simulink model "BatteryPackModel"  (R2026b)
settings: Solver=VariableStepAuto
undefined symbols (not defined in the file): Battery
settings Model: DataDictionary=VehicleData.sldd  Creator=Xu Dingyi  LastModifiedBy=29358

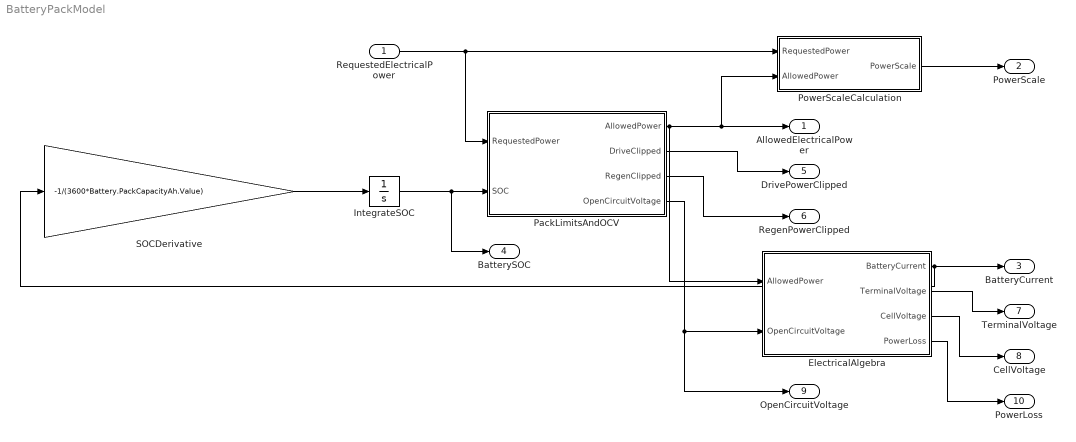
== system BatteryPackModel ==
  RequestedElectricalPower : Inport  OutDataTypeStr=double  PortDimensions=1
  ElectricalAlgebra : Subsystem
  IntegrateSOC : Integrator  InitialCondition=Battery.InitialSOC.Value  LimitOutput=on  UpperSaturationLimit=1  LowerSaturationLimit=0
  PackLimitsAndOCV : Subsystem
  PowerScaleCalculation : Subsystem
  SOCDerivative : Gain  Gain=-1/(3600*Battery.PackCapacityAh.Value)
  AllowedElectricalPower : Outport  PortDimensions=1
  PowerScale : Outport  Port=2  PortDimensions=1
  BatteryCurrent : Outport  Port=3  PortDimensions=1
  BatterySOC : Outport  Port=4  PortDimensions=1
  DrivePowerClipped : Outport  Port=5  PortDimensions=1
  RegenPowerClipped : Outport  Port=6  PortDimensions=1
  TerminalVoltage : Outport  Port=7  PortDimensions=1
  CellVoltage : Outport  Port=8  PortDimensions=1
  OpenCircuitVoltage : Outport  Port=9  PortDimensions=1
  PowerLoss : Outport  Port=10  PortDimensions=1
  wires:
  SOCDerivative/1 -> IntegrateSOC/1
  RequestedElectricalPower/1 -> PackLimitsAndOCV/1(RequestedPower), PowerScaleCalculation/1(RequestedPower)
  PackLimitsAndOCV/4(OpenCircuitVoltage) -> OpenCircuitVoltage/1, ElectricalAlgebra/2(OpenCircuitVoltage)
  PackLimitsAndOCV/3(RegenClipped) -> RegenPowerClipped/1
  PackLimitsAndOCV/2(DriveClipped) -> DrivePowerClipped/1
  PackLimitsAndOCV/1(AllowedPower) -> PowerScaleCalculation/2(AllowedPower), AllowedElectricalPower/1, ElectricalAlgebra/1(AllowedPower)
  IntegrateSOC/1 -> BatterySOC/1, PackLimitsAndOCV/2(SOC)
  PowerScaleCalculation/1(PowerScale) -> PowerScale/1
  ElectricalAlgebra/4(PowerLoss) -> PowerLoss/1
  ElectricalAlgebra/1(BatteryCurrent) -> SOCDerivative/1, BatteryCurrent/1
  ElectricalAlgebra/2(TerminalVoltage) -> TerminalVoltage/1
  ElectricalAlgebra/3(CellVoltage) -> CellVoltage/1

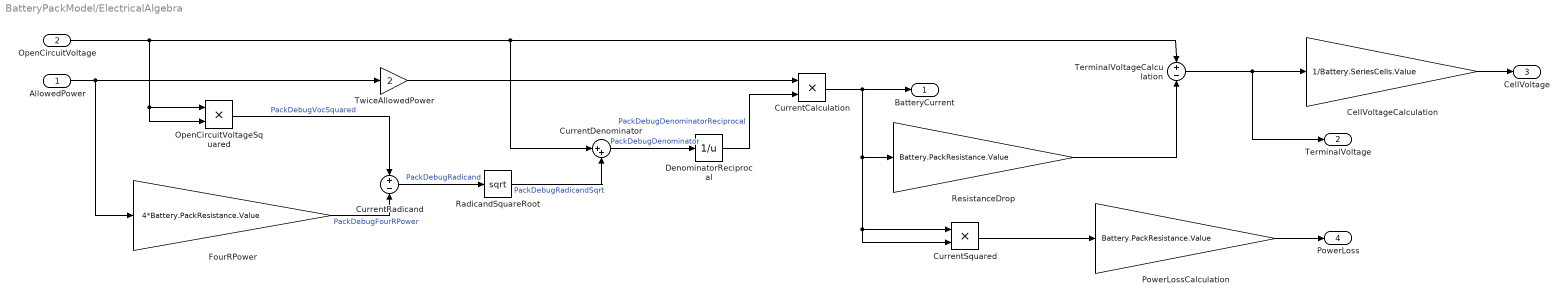
== system BatteryPackModel/ElectricalAlgebra ==
  AllowedPower : Inport
  OpenCircuitVoltage : Inport  Port=2
  CellVoltageCalculation : Gain  Gain=1/Battery.SeriesCells.Value
  CurrentCalculation : Product  Inputs=**
  CurrentDenominator : Sum  Inputs=|++
  CurrentRadicand : Sum  Inputs=+-
  CurrentSquared : Product  Inputs=**
  DenominatorReciprocal : Math  Operator=reciprocal  SignedPower=on  RndMeth=Zero
  FourRPower : Gain  Gain=4*Battery.PackResistance.Value
  OpenCircuitVoltageSquared : Product  Inputs=**
  PowerLossCalculation : Gain  Gain=Battery.PackResistance.Value
  RadicandSquareRoot : Sqrt
  ResistanceDrop : Gain  Gain=Battery.PackResistance.Value
  TerminalVoltageCalculation : Sum  Inputs=+-
  TwiceAllowedPower : Gain  Gain=2
  BatteryCurrent : Outport
  TerminalVoltage : Outport  Port=2
  CellVoltage : Outport  Port=3
  PowerLoss : Outport  Port=4
  wires:
  RadicandSquareRoot/1 -> CurrentDenominator/2  "PackDebugRadicandSqrt"
  FourRPower/1 -> CurrentRadicand/2  "PackDebugFourRPower"
  OpenCircuitVoltageSquared/1 -> CurrentRadicand/1  "PackDebugVocSquared"
  OpenCircuitVoltage/1 -> OpenCircuitVoltageSquared/2, OpenCircuitVoltageSquared/1, TerminalVoltageCalculation/1, CurrentDenominator/1
  CurrentDenominator/1 -> DenominatorReciprocal/1  "PackDebugDenominator"
  AllowedPower/1 -> TwiceAllowedPower/1, FourRPower/1
  TwiceAllowedPower/1 -> CurrentCalculation/1
  CurrentRadicand/1 -> RadicandSquareRoot/1  "PackDebugRadicand"
  DenominatorReciprocal/1 -> CurrentCalculation/2  "PackDebugDenominatorReciprocal"
  CurrentCalculation/1 -> CurrentSquared/2, CurrentSquared/1, ResistanceDrop/1, BatteryCurrent/1
  ResistanceDrop/1 -> TerminalVoltageCalculation/2
  CurrentSquared/1 -> PowerLossCalculation/1
  TerminalVoltageCalculation/1 -> TerminalVoltage/1, CellVoltageCalculation/1
  PowerLossCalculation/1 -> PowerLoss/1
  CellVoltageCalculation/1 -> CellVoltage/1

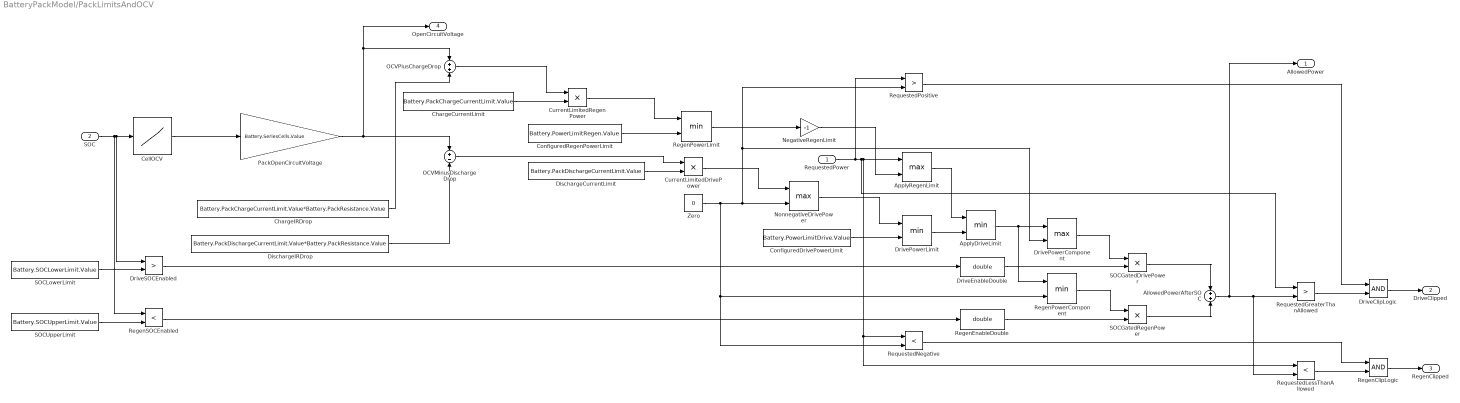
== system BatteryPackModel/PackLimitsAndOCV ==
  RequestedPower : Inport
  SOC : Inport  Port=2
  AllowedPowerAfterSOC : Sum
  ApplyDriveLimit : MinMax  Inputs=2
  ApplyRegenLimit : MinMax  Function=max  Inputs=2
  CellOCV : Lookup_n-D  NumberOfTableDimensions=1  BreakpointsForDimension1=Battery.OCVSOCBreakpoints.Value  Table=Battery.CellOCVValues.Value  ExtrapMethod=Clip  InternalRulePriority=Speed  RndMeth=Simplest
  ChargeCurrentLimit : Constant  Value=Battery.PackChargeCurrentLimit.Value
  ChargeIRDrop : Constant  Value=Battery.PackChargeCurrentLimit.Value*Battery.PackResistance.Value
  ConfiguredDrivePowerLimit : Constant  Value=Battery.PowerLimitDrive.Value
  ConfiguredRegenPowerLimit : Constant  Value=Battery.PowerLimitRegen.Value
  CurrentLimitedDrivePower : Product  Inputs=**
  CurrentLimitedRegenPower : Product  Inputs=**
  DischargeCurrentLimit : Constant  Value=Battery.PackDischargeCurrentLimit.Value
  DischargeIRDrop : Constant  Value=Battery.PackDischargeCurrentLimit.Value*Battery.PackResistance.Value
  DriveClipLogic : Logic  AllPortsSameDT=off  OutDataTypeStr=boolean
  DriveEnableDouble : DataTypeConversion  OutDataTypeStr=double
  DrivePowerComponent : MinMax  Function=max  Inputs=2
  DrivePowerLimit : MinMax  Inputs=2
  DriveSOCEnabled : RelationalOperator  Operator=>
  NegativeRegenLimit : Gain  Gain=-1
  NonnegativeDrivePower : MinMax  Function=max  Inputs=2
  OCVMinusDischargeDrop : Sum  Inputs=+-
  OCVPlusChargeDrop : Sum
  PackOpenCircuitVoltage : Gain  Gain=Battery.SeriesCells.Value
  RegenClipLogic : Logic  AllPortsSameDT=off  OutDataTypeStr=boolean
  RegenEnableDouble : DataTypeConversion  OutDataTypeStr=double
  RegenPowerComponent : MinMax  Inputs=2
  RegenPowerLimit : MinMax  Inputs=2
  RegenSOCEnabled : RelationalOperator  Operator=<
  RequestedGreaterThanAllowed : RelationalOperator  Operator=>
  RequestedLessThanAllowed : RelationalOperator  Operator=<
  RequestedNegative : RelationalOperator  Operator=<
  RequestedPositive : RelationalOperator  Operator=>
  SOCGatedDrivePower : Product  Inputs=**
  SOCGatedRegenPower : Product  Inputs=**
  SOCLowerLimit : Constant  Value=Battery.SOCLowerLimit.Value
  SOCUpperLimit : Constant  Value=Battery.SOCUpperLimit.Value
  Zero : Constant  Value=0
  AllowedPower : Outport
  DriveClipped : Outport  Port=2
  RegenClipped : Outport  Port=3
  OpenCircuitVoltage : Outport  Port=4
  wires:
  SOC/1 -> DriveSOCEnabled/1, CellOCV/1, RegenSOCEnabled/1
  DischargeCurrentLimit/1 -> CurrentLimitedDrivePower/2
  OCVMinusDischargeDrop/1 -> CurrentLimitedDrivePower/1
  CellOCV/1 -> PackOpenCircuitVoltage/1
  DrivePowerComponent/1 -> SOCGatedDrivePower/1
  SOCLowerLimit/1 -> DriveSOCEnabled/2
  ApplyDriveLimit/1 -> RegenPowerComponent/1, DrivePowerComponent/1
  CurrentLimitedDrivePower/1 -> NonnegativeDrivePower/1
  RegenSOCEnabled/1 -> RegenEnableDouble/1
  ChargeIRDrop/1 -> OCVPlusChargeDrop/2
  DriveClipLogic/1 -> DriveClipped/1
  ConfiguredRegenPowerLimit/1 -> RegenPowerLimit/2
  SOCUpperLimit/1 -> RegenSOCEnabled/2
  DriveSOCEnabled/1 -> DriveEnableDouble/1
  ChargeCurrentLimit/1 -> CurrentLimitedRegenPower/2
  PackOpenCircuitVoltage/1 -> OCVPlusChargeDrop/1, OpenCircuitVoltage/1, OCVMinusDischargeDrop/1
  SOCGatedRegenPower/1 -> AllowedPowerAfterSOC/2
  RequestedPositive/1 -> DriveClipLogic/1
  DischargeIRDrop/1 -> OCVMinusDischargeDrop/2
  OCVPlusChargeDrop/1 -> CurrentLimitedRegenPower/1
  SOCGatedDrivePower/1 -> AllowedPowerAfterSOC/1
  RegenEnableDouble/1 -> SOCGatedRegenPower/2
  RequestedNegative/1 -> RegenClipLogic/1
  CurrentLimitedRegenPower/1 -> RegenPowerLimit/1
  RegenPowerLimit/1 -> NegativeRegenLimit/1
  Zero/1 -> RegenPowerComponent/2, RequestedNegative/2, RequestedPositive/2, DrivePowerComponent/2, NonnegativeDrivePower/2
  DrivePowerLimit/1 -> ApplyDriveLimit/2
  NegativeRegenLimit/1 -> ApplyRegenLimit/2
  RequestedPower/1 -> RequestedLessThanAllowed/1, RequestedNegative/1, ApplyRegenLimit/1, RequestedGreaterThanAllowed/1, RequestedPositive/1
  RegenClipLogic/1 -> RegenClipped/1
  NonnegativeDrivePower/1 -> DrivePowerLimit/1
  ConfiguredDrivePowerLimit/1 -> DrivePowerLimit/2
  ApplyRegenLimit/1 -> ApplyDriveLimit/1
  RegenPowerComponent/1 -> SOCGatedRegenPower/1
  DriveEnableDouble/1 -> SOCGatedDrivePower/2
  AllowedPowerAfterSOC/1 -> RequestedGreaterThanAllowed/2, RequestedLessThanAllowed/2, AllowedPower/1
  RequestedGreaterThanAllowed/1 -> DriveClipLogic/2
  RequestedLessThanAllowed/1 -> RegenClipLogic/2

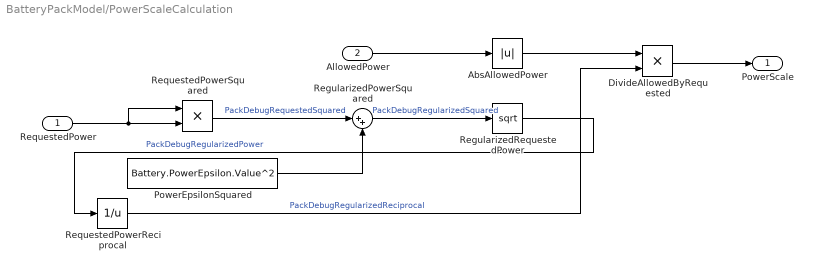
== system BatteryPackModel/PowerScaleCalculation ==
  RequestedPower : Inport
  AllowedPower : Inport  Port=2
  AbsAllowedPower : Abs
  DivideAllowedByRequested : Product  Inputs=**
  PowerEpsilonSquared : Constant  Value=Battery.PowerEpsilon.Value^2
  RegularizedPowerSquared : Sum  Inputs=|++
  RegularizedRequestedPower : Sqrt
  RequestedPowerReciprocal : Math  Operator=reciprocal  SignedPower=on  RndMeth=Zero
  RequestedPowerSquared : Product  Inputs=**
  PowerScale : Outport
  wires:
  RequestedPower/1 -> RequestedPowerSquared/1, RequestedPowerSquared/2
  RequestedPowerSquared/1 -> RegularizedPowerSquared/1  "PackDebugRequestedSquared"
  RegularizedPowerSquared/1 -> RegularizedRequestedPower/1  "PackDebugRegularizedSquared"
  PowerEpsilonSquared/1 -> RegularizedPowerSquared/2
  AllowedPower/1 -> AbsAllowedPower/1
  AbsAllowedPower/1 -> DivideAllowedByRequested/1
  DivideAllowedByRequested/1 -> PowerScale/1
  RegularizedRequestedPower/1 -> RequestedPowerReciprocal/1  "PackDebugRegularizedPower"
  RequestedPowerReciprocal/1 -> DivideAllowedByRequested/2  "PackDebugRegularizedReciprocal"
